simulink model "SWC_FDC_type"  (R2021b)
settings: Solver=FixedStepDiscrete  StartTime=0.0  StopTime=10.0  FixedStep=0.001  RelTol=1e-3
values from neighbouring files (symbols this model uses):
  DID_VCUKey = uint16(0x0202)    [vcu_local_hdr.m]
  DID_XWD = uint16(513)    [vcu_local_hdr.m]
  DIDLen_APSFunConfig = uint16(16)    [vcu_local_hdr.m]
  DIDLen_AutoLock = uint16(1)    [vcu_local_hdr.m]
  DIDLen_DKCKey = uint16(8)    [vcu_local_hdr.m]
  DIDLen_DRLDis = uint16(1)    [vcu_local_hdr.m]
  DIDLen_DynoMode = uint16(1)    [vcu_local_hdr.m]
  DIDLen_FMHTimer = uint16(1)    [vcu_local_hdr.m]
  DIDLen_LFLowPresThre = uint16(1)    [vcu_local_hdr.m]
  DIDLen_LFSensorID = uint16(4)    [vcu_local_hdr.m]
  DIDLen_LRLowPresThre = uint16(1)    [vcu_local_hdr.m]
  DIDLen_LRSensorID = uint16(4)    [vcu_local_hdr.m]
  DIDLen_RFLowPresThre = uint16(1)    [vcu_local_hdr.m]
  DIDLen_RFSensorID = uint16(4)    [vcu_local_hdr.m]
  DIDLen_RRLowPresThre = uint16(1)    [vcu_local_hdr.m]
  DIDLen_RRSensorID = uint16(4)    [vcu_local_hdr.m]
  DIDLen_SensorMode = uint16(1)    [vcu_local_hdr.m]
  DIDLen_TireSize = uint16(16)    [vcu_local_hdr.m]
  DIDLen_TPMSLearnSta = uint16(1)    [vcu_local_hdr.m]
  DIDLen_TurnLampFLThreCurr = uint16(1)    [vcu_local_hdr.m]
  DIDLen_TurnLampFRThreCurr = uint16(1)    [vcu_local_hdr.m]
  DIDLen_TurnLampRLThreCurr = uint16(1)    [vcu_local_hdr.m]
  DIDLen_TurnLampRRThreCurr = uint16(1)    [vcu_local_hdr.m]
  DIDLen_USSConfig = uint16(16)    [vcu_local_hdr.m]
  DIDLen_WhlPres = uint16(4)    [vcu_local_hdr.m]
  DIDLen_WhlSensorBattSta = uint16(1)    [vcu_local_hdr.m]
  DIDLen_WhlTmp = uint16(4)    [vcu_local_hdr.m]
  DIDLen_XWDMode = uint16(1)    [vcu_local_hdr.m]
  DIDNum_APSFunConfig = uint16(0x0903)    [vcu_local_hdr.m]
  DIDNum_AutoLock = uint16(0x0306)    [vcu_local_hdr.m]
  DIDNum_DKCKey = uint16(0x0202)    [vcu_local_hdr.m]
  DIDNum_DRLDis = uint16(0x0307)    [vcu_local_hdr.m]
  DIDNum_DynoMode = uint16(0x0203)    [vcu_local_hdr.m]
  DIDNum_FMHTimer = uint16(0x0305)    [vcu_local_hdr.m]
  DIDNum_LFLowPresThre = uint16(0x0B08)    [vcu_local_hdr.m]
  DIDNum_LFSensorID = uint16(0x0B01)    [vcu_local_hdr.m]
  DIDNum_LRLowPresThre = uint16(0x0B0A)    [vcu_local_hdr.m]
  DIDNum_LRSensorID = uint16(0x0B03)    [vcu_local_hdr.m]
  DIDNum_RFLowPresThre = uint16(0x0B09)    [vcu_local_hdr.m]
  DIDNum_RFSensorID = uint16(0x0B02)    [vcu_local_hdr.m]
  DIDNum_RRLowPresThre = uint16(0x0B0B)    [vcu_local_hdr.m]
  DIDNum_RRSensorID = uint16(0x0B04)    [vcu_local_hdr.m]
  DIDNum_SensorMode = uint16(0x0B0C)    [vcu_local_hdr.m]
  DIDNum_TireSize = uint16(0x0902)    [vcu_local_hdr.m]
  DIDNum_TPMSLearnSta = uint16(0x0B0D)    [vcu_local_hdr.m]
  DIDNum_TurnLampFLThreCurr = uint16(0x0303)    [vcu_local_hdr.m]
  DIDNum_TurnLampFRThreCurr = uint16(0x0301)    [vcu_local_hdr.m]
  DIDNum_TurnLampRLThreCurr = uint16(0x0304)    [vcu_local_hdr.m]
  DIDNum_TurnLampRRThreCurr = uint16(0x0302)    [vcu_local_hdr.m]
  DIDNum_USSConfig = uint16(0x0901)    [vcu_local_hdr.m]
  DIDNum_WhlPres = uint16(0x0B05)    [vcu_local_hdr.m]
  DIDNum_WhlSensorBattSta = uint16(0x0B07)    [vcu_local_hdr.m]
  DIDNum_WhlTmp = uint16(0x0B06)    [vcu_local_hdr.m]
  DIDNum_XWDMode = uint16(0x0201)    [vcu_local_hdr.m]
  DIDVCUKeyLength = uint16(8)    [vcu_local_hdr.m]
  ENUM_DRIVETRAIN_AWD = uint8(  2  )    [vcu_local_hdr.m]
  ENUM_DRIVETRAIN_FWD = uint8(  1  )    [vcu_local_hdr.m]
  ENUM_DRIVETRAIN_RWD = uint8(  0  )    [vcu_local_hdr.m]
  ENUM_TPMSLearnStatus_LEARNED = uint8(  1  )    [vcu_local_hdr.m]
  ENUM_TPMSLearnStatus_LEARNFAIL = uint8(  2  )    [vcu_local_hdr.m]
  ENUM_TPMSLearnStatus_NOTLEARN = uint8(  0  )    [vcu_local_hdr.m]
  ENUM_TPMSSTA_FAT = uint8(  8  )    [vcu_local_hdr.m]
  ENUM_TPMSSTA_LOWBATTERY = uint8(  2  )    [vcu_local_hdr.m]
  FALSE = boolean( 0 )    [vcu_local_hdr.m]
  ONE_INT = uint8(1)    [vcu_local_hdr.m]
  P_boolean = 0.0    [APPTypes.sldd]
  TRUE = boolean( 1 )    [vcu_local_hdr.m]
  ZERO_FLOAT = single(0)    [vcu_local_hdr.m]
  ZERO_INT = uint8(0)    [vcu_local_hdr.m]
undefined symbols (not defined in the file or in its folder): f32_ApsOutVehSpdSig, KHAL_DKCDecryptEnable_flg_ovrdflg, KHAL_DKCDecryptEnable_flg_ovrdval, KHAL_RandomNumberY1_enum, KHAL_RandomNumberY2_enum, KHAL_RandomNumberY_ovrdflg, KHAL_TPMSRESBUTT_flg_ovrdflg, KHAL_TPMSRESBUTT_flg_ovrdval, R_DIDWriteCDD_CSOP_DIDSet_APSFunConfig, R_DIDWriteCDD_CSOP_DIDSet_AutoLock, R_DIDWriteCDD_CSOP_DIDSet_DKCKey, R_DIDWriteCDD_CSOP_DIDSet_DRLDis, R_DIDWriteCDD_CSOP_DIDSet_DynoMode, R_DIDWriteCDD_CSOP_DIDSet_FMHTimer, R_DIDWriteCDD_CSOP_DIDSet_LFLowPresThre, R_DIDWriteCDD_CSOP_DIDSet_LFSensorID, R_DIDWriteCDD_CSOP_DIDSet_LRLowPresThre, R_DIDWriteCDD_CSOP_DIDSet_LRSensorID, R_DIDWriteCDD_CSOP_DIDSet_RFLowPresThre, R_DIDWriteCDD_CSOP_DIDSet_RFSensorID, R_DIDWriteCDD_CSOP_DIDSet_RRLowPresThre, R_DIDWriteCDD_CSOP_DIDSet_RRSensorID, R_DIDWriteCDD_CSOP_DIDSet_SensorMode, R_DIDWriteCDD_CSOP_DIDSet_TireSize, R_DIDWriteCDD_CSOP_DIDSet_TPMSLearnSta, R_DIDWriteCDD_CSOP_DIDSet_TurnLampFLThreCurr, R_DIDWriteCDD_CSOP_DIDSet_TurnLampFRThreCurr, R_DIDWriteCDD_CSOP_DIDSet_TurnLampRLThreCurr, R_DIDWriteCDD_CSOP_DIDSet_TurnLampRRThreCurr, R_DIDWriteCDD_CSOP_DIDSet_USSConfig, R_DIDWriteCDD_CSOP_DIDSet_WhlPres, R_DIDWriteCDD_CSOP_DIDSet_WhlSensorBattSta, R_DIDWriteCDD_CSOP_DIDSet_WhlTmp, R_DIDWriteCDD_CSOP_DIDSet_XWDMode, R_E2E_CAN3_VCU1_CSOP_Write_CAN3_VCU1, R_E2E_CAN3_VCU1_toNIDEC_CSOP_Write_CAN3_VCU1_toNIDEC, R_E2E_CAN4_VCU1_CSOP_Write_CAN4_VCU1, R_FDCCDD_Inner_CSOP_FDC_AppCallSleep, R_HALINCDD_CSOP_PAS_Handler, R_HALINCDD_CSOP_UDS_Main, R_HALOUT_APS_CSOP_ApsOutput, R_HALOUTCDD_CSOP_AppNmStateReq, R_HALOUTCDD_CSOP_SetAcoreRebootCmdACK, R_HALOUTCDD_CSOP_SetSysPwrStat, R_HALOUTCDD_CSOP_SleepRequest, R_IOExpOUT_CDD_CSOP_IOExpSetVal, R_J1939_CAN1_CFGEM1_BAM_CSOP_Write_CAN1_CFGEM1_BAM, R_J1939_CAN1_CFGEM1_DT_CSOP_Write_CAN1_CFGEM1_DT, R_NVMReadCDD_Inner_NVM_ReadOperation, R_NVMWriteCDD_Inner_NVM_WriteOperation, R_UDSCDD_CSOP_DdmRestartOperationCycle, R_WDGCDD_CSOP_Call_Watchdog, R_WDGCDD_CSOP_Call_WDG_AppEnd, R_WDGCDD_CSOP_Call_WDG_AppStart, u16_DIDLen_APSFunConfig, u16_DIDLen_AutoLock, u16_DIDLen_DKCKey, u16_DIDLen_DRLDis, u16_DIDLen_DynoMode, u16_DIDLen_FMHTimer ... (+83)
libraries: simulink x215, FVT_lib x143, hcu_lib x19, hdlsllib x9, app x1, halin x1, halout x1, inp x1, outp x1
(part 4 of 13)

== system SWC_FDC_type/run_SWC_FDC_RxTx_5ms_sys/Subsystem3 ==
  BOUTP_outputs : Inport
  Enable : EnablePort
  Bus Selector3 : BusSelector  OutputSignals=VOUTP_PowerSta_enum,VOUTP_BrkPedalPos_pct,VOUTP_ActAPSPosn_pct,VOUTP_LFRawWhlSpeed_kph,VOUTP_RFRawWhlSpeed_kph,VOUTP_LRRawWhlSpeed_kph,VOUTP_RRRawWhlSpeed_kph,VOUTP_LFRawWhlSpeedV_flg,VOUTP_RFRawWhlSpeedV_flg,VOUTP_LRRawWhlSpeedV_flg,VOUTP_RRRawWhlSpeedV_flg,VOUTP_LFWhlRotDir_enum,VOUTP_RFWhlRotDir_enum,VOUTP_LRWhlRotDir_enum,VOUTP_RRWhlRotDir_enum,VOUTP_LFPulseCountV_flg,VOUTP_RFPulseCountV_flg,VOUTP_LRPulseCountV_flg,VOUTP_RRPulseCountV_flg,VOUTP_LFPulseCount_enum,VOUTP_RFPulseCount_enum,VOUTP_LRPulseCount_enum,VOUTP_RRPulseCount_enum,VOUTP_VehSpeedToAPM_kph,VOUTP_APSCtrlAvail_flg,VOUTP_ShifterHandleCmd_enum,VOUTP_DriIntend_enum,VOUTP_EPSAOIControl_enum,VOUTP_SASAngle_Deg,VOUTP_SASSpeed_degps,VOUTP_SASSpeedValid_flg,VOUTP_SASCAL_flg,VOUTP_SASV_flg,VOUTP_GRADE_Deg,VOUTP_YawRate_degps,VOUTP_LatAccel_Gps,VOUTP_LongAccel_Gps,VOUTP_MCPressure_bar,VOUTP_YawRateV_flg,VOUTP_LatAccelV_flg,VOUTP_LongAccelV_flg,VOUTP_MCPressureV_bar,VOUTP_BrkSwSta_flg,VOUTP_BrkSwV_flg,VOUTP_ESCStandstill_flg,VOUTP_ESCAPSSta_enum,VOUTP_EPBExtReleaseAvail_flg,VOUTP_EPBExtApplyAvail_flg,VOUTP_EPBErrSta_enum,VOUTP_EPBSta_enum,VOUTP_AVMparkingcancel_enum,VOUTP_AVMparkingexcute_enum,VOUTP_AVMParkingmode_enum,VOUTP_AVMErrSTA_flg,VOUTP_IVIStatus_flg,VOUTP_CAASSw_enum,VOUTP_IVIScreen_enum,VOUTP_VehSpeedToAPM_kph,VOUTP_ABSActive_flg,VOUTP_TCSActiveToAPM_flg,VOUTP_DriverSeatBeltCmd_flg,VOUTP_RFPressIndi_enum,VOUTP_LFPressIndi_enum,VOUTP_RRPressIndi_enum,VOUTP_LRPressIndi_enum,VOUTP_sigAmbAirT_C,VOUTP_VehSpeedToAPM_kph,VOUTP_VehSpeedToAPM_kph
  Bus Selector4 : BusSelector  OutputSignals=VOUTP_BrkPedalPosTimeOut_flg,VOUTP_LFRawWhlSpeedTimeOut_flg,VOUTP_RFRawWhlSpeedTimeOut_flg,VOUTP_LRRawWhlSpeedTimeOut_flg,VOUTP_RRRawWhlSpeedTimeOut_flg,VOUTP_LFRawWhlSpeedVTimeOut_flg,VOUTP_RFRawWhlSpeedVTimeOut_flg,VOUTP_LRRawWhlSpeedVTimeOut_flg,VOUTP_RRRawWhlSpeedVTimeOut_flg,VOUTP_LFWhlRotDirTimeOut_flg,VOUTP_RFWhlRotDirTimeOut_flg,VOUTP_LRWhlRotDirTimeOut_flg,VOUTP_RRWhlRotDirTimeOut_flg,VOUTP_LFPulseCountVTimeOut_flg,VOUTP_RFPulseCountVTimeOut_flg,VOUTP_LRPulseCountVTimeOut_flg,VOUTP_RRPulseCountVTimeOut_flg,VOUTP_LFPulseCountTimeOut_flg,VOUTP_RFPulseCountTimeOut_flg,VOUTP_LRPulseCountTimeOut_flg,VOUTP_RRPulseCountTimeOut_flg,VOUTP_ShifterHandleCmdTimeOut_flg,VOUTP_DriIntendTimeOut_flg,VOUTP_EPSAOIControlTimeOut_flg,VOUTP_SASAngleTimeOut_flg,VOUTP_SASSpeedTimeOut_flg,VOUTP_SASSpeedValidTimeOut_flg,VOUTP_SASCALTimeOut_flg,VOUTP_SASVTimeOut_flg,VOUTP_GRADETimeOut_flg,VOUTP_YawRateTimeOut_flg,VOUTP_LatAccelTimeOut_flg,VOUTP_LongAccelTimeOut_flg,VOUTP_MCPressureTimeOut_flg,VOUTP_YawRateVTimeOut_flg,VOUTP_LatAccelVTimeOut_flg,VOUTP_LongAccelVTimeOut_flg,VOUTP_MCPressureVTimeOut_flg,VOUTP_BrkSwStaTimeOut_flg,VOUTP_BrkSwVTimeOut_flg,VOUTP_ESCStandstillTimeOut_flg,VOUTP_ESCAPSStaTimeOut_flg,VOUTP_EPBExtReleaseAvailTimeOut_flg,VOUTP_EPBExtApplyAvailTimeOut_flg,VOUTP_EPBErrStaTimeOut_flg,VOUTP_EPBStaTimeOut_flg,VOUTP_AVMparkingcancelTimeOut_flg,VOUTP_AVMparkingexcuteTimeOut_flg,VOUTP_AVMParkingmodeTimeOut_flg,VOUTP_AVMErrSTATimeOut_flg,VOUTP_IVIStatusTimeOut_flg,VOUTP_CAASSwTimeOut_flg,VOUTP_IVIScreenTimeOut_flg,VOUTP_ABSActiveTimeOut_flg,VOUTP_TCSActiveTimeOut_flg,VOUTP_DriverSeatBeltCmdTimeOut_flg,VOUTP_RFPressIndi_enum,VOUTP_LFPressIndi_enum,VOUTP_RRPressIndi_enum,VOUTP_LRPressIndi_enum,VOUTP_sigAmbAirT_C
  Data Type Conversion{6..13,17..19,21..96,98..106,123} (97 alike) : DataTypeConversion  OutDataTypeStr=uint8
  Data Type Conversion{14..16,20} (4 alike) : DataTypeConversion  OutDataTypeStr=int16
  Data Type Conversion4 : DataTypeConversion  OutDataTypeStr=single
  Ground{,1..10} (11 alike) : Ground
  R_HALOUT_APS_CSOP_ApsSetData : FunctionCaller  FunctionPrototype=R_HALOUT_APS_CSOP_ApsSetData(u8_SetPwrSta,f32_SetBrkPedalPos,f32_SetActAPSPosn,f32_SetLF_RawWhlSpeed,f32_SetRF_RawWhlSpeed,f32_SetLR_RawWhlSpeed,f32_SetRR_RawWhlSpeed,u8_SetLF_RawWhlSpeed_V,u8_SetRF_RawWhlSpeed_V,u8_SetLR_RawWhlSpeed_V,u8_SetRR_RawWhlSpeed_V,u8_SetLF_WhlRotDir,u8_SetRF_WhlRotDir,u8_SetLR_WhlRotDir,u8_SetRR_WhlRotDir,u8_SetLF_PulseCount_V,u8_SetRF_PulseCount_V,u8_SetLR_PulseCount_V,u8_SetRR_PulseCount_V,s16_SetLF_PulseCount,s16_SetRF_PulseCount,s16_SetLR_PulseCount,s16_SetRR_PulseCount,u8_SetAPS_Active,u8_SetAPS_CtrlAvail,u8_SetShifter_Handle_Cmd,u8_SetDriIntend,u8_SetEPS_AOI_Control,f32_SetSAS_Angle,f32_SetSAS_Speed,u8_SetSAS_Speed_Valid,u8_SetSAS_CAL,u8_SetSAS_OK,f32_SetGRADE,f32_SetYawRate,f32_SetLatAccel,f32_SetLongAccel,f32_SetMCPressure,u8_SetYawRate_V,u8_SetLatAccel_V,u8_SetLongAccel_V,u8_SetMCPressure_V,u8_SetBrkSw_Sta,u8_SetBrkSw_V,u8_SetESC_Standstill,u8_SetESC_APS_Sta,u8_SetEPBExtReleaseAvail,u8_SetEPBExtApplyAvail,u8_SetEPBErrSta,u8_SetEPBSta,u8_SetAllDoorSW,u8_SetHoodSW,u8_SetTailgate_SW,u8_SetAVM_parking_cancel,u8_SetAVM_parking_excute,u8_SetAVM_Parking_mode,u8_SetAVM_Err_STA,u8_SetIVI_Status,u8_SetCAAS_Sw,u8_SetIVI_Screen,u8_SetCAAS_CtrlAvail,u8_SetABS_Active,u8_SetTCS_Active,u8_SetDriverSeatBeltCmd,u8_SetDrDoorSW,u8_SetPsDoorSW,u8_SetRLDoorSW,u8_SetRRDoorSW,u8_SetRFPressIndi,u8_SetLFPressIndi,u8_SetRRPressIndi,u8_SetLRPressIndi,f32_SetsigAmbAirT,f32_SetVehActSpd,u8_SetCAAS_Active)  InputArgumentSpecifications=uint8(1), single(1), single(1), single(1), single(1), single(1), single(1), uint8(1), uint8(1), uint8(1), uint8(1), uint8(1), uint8(1), uint8(1), uint8(1), uint8(1), uint8(1), uint8(1), uint8(1), int16(1), int16(1), int16(1), int16(1), uint8(1), uint8(1), uint8(1), uint8(1), uint8(1), single(1), single(1), uint8(1), uint8(1), uint8(1), single(1), single(1), single(1), single(1), single(1), uint8(1), uint8(1), uint8(1), uint8(1), uint8(1), uint8(1), uint8(1), uint8(1), uint8(1), uint8(1), uint8(1), uint8(1), uint8(1), uint8(1), uint8(1), uint8(1), uint8(1), uint8(1), uint8(1), uint8(1), uint8(1), uint8(1), uint8(1), uint8(1), uint8(1), uint8(1), uint8(1), uint8(1), uint8(1), uint8(1), uint8(1), uint8(1), uint8(1), uint8(1), single(1), single(1), uint8(1)
  R_HALOUT_APS_CSOP_ApsSetTimeout : FunctionCaller  FunctionPrototype=R_HALOUT_APS_CSOP_ApsSetTimeout(u8_SetBrkPedalPosTO,u8_SetLF_RawWhlSpeedTO,u8_SetRF_RawWhlSpeedTO,u8_SetLR_RawWhlSpeedTO,u8_SetRR_RawWhlSpeedTO,u8_SetLF_RawWhlSpeed_VTO,u8_SetRF_RawWhlSpeed_VTO,u8_SetLR_RawWhlSpeed_VTO,u8_SetRR_RawWhlSpeed_VTO,u8_SetLF_WhlRotDirTO,u8_SetRF_WhlRotDirTO,u8_SetLR_WhlRotDirTO,u8_SetRR_WhlRotDirTO,u8_SetLF_PulseCount_VTO,u8_SetRF_PulseCount_VTO,u8_SetLR_PulseCount_VTO,u8_SetRR_PulseCount_VTO,u8_SetLF_PulseCountTO,u8_SetRF_PulseCountTO,u8_SetLR_PulseCountTO,u8_SetRR_PulseCountTO,u8_SetShifter_Handle_CmdTO,u8_SetDriIntendTO,u8_SetEPS_AOI_ControlTO,u8_SetSAS_AngleTO,u8_SetSAS_SpeedTO,u8_SetSAS_Speed_ValidTO,u8_SetSAS_CALTO,u8_SetSAS_OKTO,u8_SetGRADETO,u8_SetYawRateTO,u8_SetLatAccelTO,u8_SetLongAccelTO,u8_SetMCPressureTO,u8_SetYawRate_VTO,u8_SetLatAccel_VTO,u8_SetLongAccel_VTO,u8_SetMCPressure_VTO,u8_SetBrkSw_StaTO,u8_SetBrkSw_VTO,u8_SetESC_StandstillTO,u8_SetESC_APS_StaTO,u8_SetEPBExtReleaseAvailTO,u8_SetEPBExtApplyAvailTO,u8_SetEPBErrStaTO,u8_SetEPBStaTO,u8_SetAVM_parking_cancelTO,u8_SetAVM_parking_excuteTO,u8_SetAVM_Parking_modeTO,u8_SetAVM_Err_STATO,u8_SetIVI_StatusTO,u8_SetCAAS_SwTO,u8_SetIVI_ScreenTO,u8_SetABS_ActiveTO,u8_SetTCS_ActiveTO,u8_SetDriverSeatBeltCmdTO,u8_SetRFPressIndiTO,u8_SetLFPressIndiTO,u8_SetRRPressIndiTO,u8_SetLRPressIndiTO,u8_SetsigAmbAirTTO)  InputArgumentSpecifications=uint8(1), uint8(1), uint8(1), uint8(1), uint8(1), uint8(1), uint8(1), uint8(1), uint8(1), uint8(1), uint8(1), uint8(1), uint8(1), uint8(1), uint8(1), uint8(1), uint8(1), uint8(1), uint8(1), uint8(1), uint8(1), uint8(1), uint8(1), uint8(1), uint8(1), uint8(1), uint8(1), uint8(1), uint8(1), uint8(1), uint8(1), uint8(1), uint8(1), uint8(1), uint8(1), uint8(1), uint8(1), uint8(1), uint8(1), uint8(1), uint8(1), uint8(1), uint8(1), uint8(1), uint8(1), uint8(1), uint8(1), uint8(1), uint8(1), uint8(1), uint8(1), uint8(1), uint8(1), uint8(1), uint8(1), uint8(1), uint8(1), uint8(1), uint8(1), uint8(1), uint8(1)
  Terminator{1..9} (9 alike) : Terminator
  wires:
  Data Type Conversion75/1 -> R_HALOUT_APS_CSOP_ApsSetTimeout/33
  Bus Selector4/29 -> Data Type Conversion61/1  "<VOUTP_SASVTimeOut_flg>"
  Bus Selector3/45 -> Data Type Conversion30/1  "<VOUTP_ESCStandstill_flg>"
  Bus Selector4/41 -> Data Type Conversion73/1  "<VOUTP_ESCStandstillTimeOut_flg>"
  Data Type Conversion51/1 -> R_HALOUT_APS_CSOP_ApsSetTimeout/19
  Bus Selector4/1 -> Data Type Conversion80/1  "<VOUTP_BrkPedalPosTimeOut_flg>"
  Bus Selector4/10 -> Data Type Conversion42/1  "<VOUTP_LFWhlRotDirTimeOut_flg>"
  Data Type Conversion84/1 -> R_HALOUT_APS_CSOP_ApsSetTimeout/55
  Bus Selector3/48 -> Data Type Conversion32/1  "<VOUTP_EPBExtApplyAvail_flg>"
  Bus Selector3/43 -> Data Type Conversion28/1  "<VOUTP_BrkSwSta_flg>"
  Bus Selector3/56 -> R_HALOUT_APS_CSOP_ApsSetData/59  "<VOUTP_CAASSw_enum>"
  Bus Selector4/39 -> Data Type Conversion71/1  "<VOUTP_BrkSwStaTimeOut_flg>"
  Bus Selector3/39 -> Data Type Conversion24/1  "<VOUTP_YawRateV_flg>"
  Data Type Conversion123/1 -> R_HALOUT_APS_CSOP_ApsSetTimeout/2
  Bus Selector3/21 -> Data Type Conversion14/1  "<VOUTP_RFPulseCount_enum>"
  Bus Selector3/67 -> Terminator8/1  "<VOUTP_VehSpeedToAPM_kph>"
  Bus Selector3/54 -> Data Type Conversion36/1  "<VOUTP_AVMErrSTA_flg>"
  Bus Selector3/47 -> Data Type Conversion31/1  "<VOUTP_EPBExtReleaseAvail_flg>"
  Data Type Conversion82/1 -> R_HALOUT_APS_CSOP_ApsSetTimeout/47
  Bus Selector4/34 -> Data Type Conversion66/1  "<VOUTP_MCPressureTimeOut_flg>"
  Bus Selector4/42 -> Data Type Conversion76/1  "<VOUTP_ESCAPSStaTimeOut_flg>"
  Data Type Conversion85/1 -> R_HALOUT_APS_CSOP_ApsSetTimeout/49
  Bus Selector4/8 -> Data Type Conversion44/1  "<VOUTP_LRRawWhlSpeedVTimeOut_flg>"
  Bus Selector4/9 -> Data Type Conversion41/1  "<VOUTP_RRRawWhlSpeedVTimeOut_flg>"
  Bus Selector3/55 -> Data Type Conversion37/1  "<VOUTP_IVIStatus_flg>"
  Bus Selector4/46 -> Data Type Conversion79/1  "<VOUTP_EPBStaTimeOut_flg>"
  Bus Selector3/15 -> R_HALOUT_APS_CSOP_ApsSetData/15  "<VOUTP_RRWhlRotDir_enum>"
  Data Type Conversion35/1 -> R_HALOUT_APS_CSOP_ApsSetData/53
  Bus Selector4/37 -> Data Type Conversion69/1  "<VOUTP_LongAccelVTimeOut_flg>"
  Bus Selector4/17 -> Data Type Conversion49/1  "<VOUTP_RRPulseCountVTimeOut_flg>"
  Bus Selector3/34 -> R_HALOUT_APS_CSOP_ApsSetData/34  "<VOUTP_GRADE_Deg>"
  Ground9/1 -> Data Type Conversion96/1
  Bus Selector4/5 -> Data Type Conversion38/1  "<VOUTP_RRRawWhlSpeedTimeOut_flg>"
  Bus Selector4/2 -> Data Type Conversion123/1  "<VOUTP_LFRawWhlSpeedTimeOut_flg>"
  Data Type Conversion89/1 -> R_HALOUT_APS_CSOP_ApsSetTimeout/56
  Bus Selector4/11 -> Data Type Conversion43/1  "<VOUTP_RFWhlRotDirTimeOut_flg>"
  Bus Selector4/19 -> Data Type Conversion51/1  "<VOUTP_RFPulseCountTimeOut_flg>"
  Data Type Conversion60/1 -> R_HALOUT_APS_CSOP_ApsSetTimeout/27
  Data Type Conversion64/1 -> R_HALOUT_APS_CSOP_ApsSetTimeout/28
  Bus Selector3/20 -> Data Type Conversion20/1  "<VOUTP_LFPulseCount_enum>"
  Data Type Conversion21/1 -> R_HALOUT_APS_CSOP_ApsSetData/31
  Bus Selector4/33 -> Data Type Conversion75/1  "<VOUTP_LongAccelTimeOut_flg>"
  Bus Selector4/26 -> Data Type Conversion59/1  "<VOUTP_SASSpeedTimeOut_flg>"
  Data Type Conversion63/1 -> R_HALOUT_APS_CSOP_ApsSetTimeout/31
  Bus Selector4/40 -> Data Type Conversion72/1  "<VOUTP_BrkSwVTimeOut_flg>"
  Bus Selector4/56 -> Data Type Conversion89/1  "<VOUTP_DriverSeatBeltCmdTimeOut_flg>"
  Bus Selector4/48 -> Data Type Conversion83/1  "<VOUTP_AVMparkingexcuteTimeOut_flg>"
  Bus Selector4/6 -> Data Type Conversion39/1  "<VOUTP_LFRawWhlSpeedVTimeOut_flg>"
  Data Type Conversion26/1 -> R_HALOUT_APS_CSOP_ApsSetData/41
  Bus Selector4/60 -> Terminator4/1  "<VOUTP_LRPressIndi_enum>"
  Bus Selector4/51 -> Data Type Conversion86/1  "<VOUTP_IVIStatusTimeOut_flg>"
  Data Type Conversion103/1 -> R_HALOUT_APS_CSOP_ApsSetData/63
  Bus Selector4/57 -> Terminator1/1  "<VOUTP_RFPressIndi_enum>"
  Ground5/1 -> Data Type Conversion106/1
  Ground1/1 -> Data Type Conversion91/1
  Bus Selector4/27 -> Data Type Conversion60/1  "<VOUTP_SASSpeedValidTimeOut_flg>"
  Bus Selector3/66 -> R_HALOUT_APS_CSOP_ApsSetData/73  "<VOUTP_sigAmbAirT_C>"
  Data Type Conversion87/1 -> R_HALOUT_APS_CSOP_ApsSetTimeout/52
  Bus Selector4/13 -> Data Type Conversion55/1  "<VOUTP_RRWhlRotDirTimeOut_flg>"
  Data Type Conversion24/1 -> R_HALOUT_APS_CSOP_ApsSetData/39
  Data Type Conversion61/1 -> R_HALOUT_APS_CSOP_ApsSetTimeout/29
  Bus Selector4/7 -> Data Type Conversion40/1  "<VOUTP_RFRawWhlSpeedVTimeOut_flg>"
  Bus Selector4/35 -> Data Type Conversion67/1  "<VOUTP_YawRateVTimeOut_flg>"
  Bus Selector4/25 -> Data Type Conversion58/1  "<VOUTP_SASAngleTimeOut_flg>"
  Bus Selector3/49 -> R_HALOUT_APS_CSOP_ApsSetData/49  "<VOUTP_EPBErrSta_enum>"
  Data Type Conversion76/1 -> R_HALOUT_APS_CSOP_ApsSetTimeout/42
  Bus Selector4/55 -> Data Type Conversion84/1  "<VOUTP_TCSActiveTimeOut_flg>"
  Ground4/1 -> Data Type Conversion94/1
  Data Type Conversion39/1 -> R_HALOUT_APS_CSOP_ApsSetTimeout/6
  Bus Selector4/45 -> Data Type Conversion78/1  "<VOUTP_EPBErrStaTimeOut_flg>"
  Bus Selector4/12 -> Data Type Conversion45/1  "<VOUTP_LRWhlRotDirTimeOut_flg>"
  Bus Selector4/24 -> Data Type Conversion57/1  "<VOUTP_EPSAOIControlTimeOut_flg>"
  Data Type Conversion11/1 -> R_HALOUT_APS_CSOP_ApsSetData/17
  Bus Selector3/42 -> Data Type Conversion27/1  "<VOUTP_MCPressureV_bar>"
  Bus Selector4/20 -> Data Type Conversion52/1  "<VOUTP_LRPulseCountTimeOut_flg>"
  Bus Selector3/23 -> Data Type Conversion16/1  "<VOUTP_RRPulseCount_enum>"
  Bus Selector4/54 -> Data Type Conversion81/1  "<VOUTP_ABSActiveTimeOut_flg>"
  Bus Selector4/49 -> Data Type Conversion85/1  "<VOUTP_AVMParkingmodeTimeOut_flg>"
  Bus Selector4/22 -> Data Type Conversion56/1  "<VOUTP_ShifterHandleCmdTimeOut_flg>"
  Bus Selector4/38 -> Data Type Conversion74/1  "<VOUTP_MCPressureVTimeOut_flg>"
  Bus Selector4/50 -> Data Type Conversion95/1  "<VOUTP_AVMErrSTATimeOut_flg>"
  Bus Selector4/23 -> Data Type Conversion70/1  "<VOUTP_DriIntendTimeOut_flg>"
  Data Type Conversion25/1 -> R_HALOUT_APS_CSOP_ApsSetData/40
  Data Type Conversion92/1 -> R_HALOUT_APS_CSOP_ApsSetTimeout/60
  Bus Selector4/36 -> Data Type Conversion68/1  "<VOUTP_LatAccelVTimeOut_flg>"
  Bus Selector4/18 -> Data Type Conversion54/1  "<VOUTP_LFPulseCountTimeOut_flg>"
  Bus Selector4/15 -> Data Type Conversion47/1  "<VOUTP_RFPulseCountVTimeOut_flg>"
  Data Type Conversion9/1 -> R_HALOUT_APS_CSOP_ApsSetData/11
  Data Type Conversion10/1 -> R_HALOUT_APS_CSOP_ApsSetData/16
  Bus Selector4/21 -> Data Type Conversion53/1  "<VOUTP_RRPulseCountTimeOut_flg>"
  Bus Selector4/28 -> Data Type Conversion64/1  "<VOUTP_SASCALTimeOut_flg>"
  Data Type Conversion77/1 -> R_HALOUT_APS_CSOP_ApsSetTimeout/44
  Data Type Conversion23/1 -> R_HALOUT_APS_CSOP_ApsSetData/33
  Data Type Conversion93/1 -> R_HALOUT_APS_CSOP_ApsSetTimeout/59
  Data Type Conversion69/1 -> R_HALOUT_APS_CSOP_ApsSetTimeout/37
  Data Type Conversion46/1 -> R_HALOUT_APS_CSOP_ApsSetTimeout/14
  Data Type Conversion74/1 -> R_HALOUT_APS_CSOP_ApsSetTimeout/38
  Bus Selector3/25 -> Data Type Conversion18/1  "<VOUTP_APSCtrlAvail_flg>"
  Data Type Conversion62/1 -> R_HALOUT_APS_CSOP_ApsSetTimeout/30
  Data Type Conversion52/1 -> R_HALOUT_APS_CSOP_ApsSetTimeout/20
  Data Type Conversion71/1 -> R_HALOUT_APS_CSOP_ApsSetTimeout/39
  Data Type Conversion80/1 -> R_HALOUT_APS_CSOP_ApsSetTimeout/1
  Data Type Conversion43/1 -> R_HALOUT_APS_CSOP_ApsSetTimeout/11
  Bus Selector3/37 -> R_HALOUT_APS_CSOP_ApsSetData/37  "<VOUTP_LongAccel_Gps>"
  Bus Selector3/31 -> Data Type Conversion21/1  "<VOUTP_SASSpeedValid_flg>"
  Data Type Conversion86/1 -> R_HALOUT_APS_CSOP_ApsSetTimeout/51
  Data Type Conversion65/1 -> R_HALOUT_APS_CSOP_ApsSetTimeout/32
  Bus Selector3/53 -> R_HALOUT_APS_CSOP_ApsSetData/56  "<VOUTP_AVMParkingmode_enum>"
  Data Type Conversion32/1 -> R_HALOUT_APS_CSOP_ApsSetData/48
  Data Type Conversion106/1 -> R_HALOUT_APS_CSOP_ApsSetTimeout/57
  Bus Selector3/28 -> R_HALOUT_APS_CSOP_ApsSetData/28  "<VOUTP_EPSAOIControl_enum>"
  Data Type Conversion91/1 -> R_HALOUT_APS_CSOP_ApsSetTimeout/61
  Data Type Conversion70/1 -> R_HALOUT_APS_CSOP_ApsSetTimeout/23
  Data Type Conversion102/1 -> R_HALOUT_APS_CSOP_ApsSetData/64
  Data Type Conversion22/1 -> R_HALOUT_APS_CSOP_ApsSetData/32
  Data Type Conversion58/1 -> R_HALOUT_APS_CSOP_ApsSetTimeout/25
  Data Type Conversion66/1 -> R_HALOUT_APS_CSOP_ApsSetTimeout/34
  Data Type Conversion95/1 -> R_HALOUT_APS_CSOP_ApsSetTimeout/50
  Data Type Conversion42/1 -> R_HALOUT_APS_CSOP_ApsSetTimeout/10
  Data Type Conversion94/1 -> R_HALOUT_APS_CSOP_ApsSetTimeout/58
  Bus Selector4/30 -> Data Type Conversion62/1  "<VOUTP_GRADETimeOut_flg>"
  Data Type Conversion48/1 -> R_HALOUT_APS_CSOP_ApsSetTimeout/16
  Data Type Conversion81/1 -> R_HALOUT_APS_CSOP_ApsSetTimeout/54
  Data Type Conversion83/1 -> R_HALOUT_APS_CSOP_ApsSetTimeout/48
  Data Type Conversion15/1 -> R_HALOUT_APS_CSOP_ApsSetData/22
  Bus Selector3/16 -> Data Type Conversion10/1  "<VOUTP_LFPulseCountV_flg>"
  [BOUTP_outputs] -> Bus Selector3/1
  Bus Selector3/59 -> Data Type Conversion104/1  "<VOUTP_ABSActive_flg>"
  Bus Selector3/10 -> Data Type Conversion8/1  "<VOUTP_LRRawWhlSpeedV_flg>"
  Bus Selector3/51 -> R_HALOUT_APS_CSOP_ApsSetData/54  "<VOUTP_AVMparkingcancel_enum>"
  Bus Selector3/17 -> Data Type Conversion11/1  "<VOUTP_RFPulseCountV_flg>"
  Bus Selector3/14 -> R_HALOUT_APS_CSOP_ApsSetData/14  "<VOUTP_LRWhlRotDir_enum>"
  Ground6/1 -> Data Type Conversion17/1
  Data Type Conversion30/1 -> R_HALOUT_APS_CSOP_ApsSetData/45
  Bus Selector3/68 -> Terminator9/1  "<VOUTP_VehSpeedToAPM_kph>"
  Ground7/1 -> Data Type Conversion105/1
  Data Type Conversion55/1 -> R_HALOUT_APS_CSOP_ApsSetTimeout/13
  Bus Selector3/18 -> Data Type Conversion12/1  "<VOUTP_LRPulseCountV_flg>"
  Bus Selector3/41 -> Data Type Conversion26/1  "<VOUTP_LongAccelV_flg>"
  Bus Selector3/1 -> R_HALOUT_APS_CSOP_ApsSetData/1  "<VOUTP_PowerSta_enum>"
  Data Type Conversion8/1 -> R_HALOUT_APS_CSOP_ApsSetData/10
  Bus Selector3/60 -> Data Type Conversion103/1  "<VOUTP_TCSActiveToAPM_flg>"
  Bus Selector3/19 -> Data Type Conversion13/1  "<VOUTP_RRPulseCountV_flg>"
  Bus Selector3/32 -> Data Type Conversion22/1  "<VOUTP_SASCAL_flg>"
  Ground2/1 -> Data Type Conversion92/1
  Bus Selector4/3 -> Data Type Conversion50/1  "<VOUTP_RFRawWhlSpeedTimeOut_flg>"
  Data Type Conversion54/1 -> R_HALOUT_APS_CSOP_ApsSetTimeout/18
  Bus Selector4/47 -> Data Type Conversion82/1  "<VOUTP_AVMparkingcancelTimeOut_flg>"
  Bus Selector4/31 -> Data Type Conversion63/1  "<VOUTP_YawRateTimeOut_flg>"
  [BOUTP_outputs] -> Bus Selector4/1
  Bus Selector3/62 -> R_HALOUT_APS_CSOP_ApsSetData/69  "<VOUTP_RFPressIndi_enum>"
  Ground3/1 -> Data Type Conversion93/1
  Bus Selector4/14 -> Data Type Conversion46/1  "<VOUTP_LFPulseCountVTimeOut_flg>"
  Bus Selector4/16 -> Data Type Conversion48/1  "<VOUTP_LRPulseCountVTimeOut_flg>"
  Bus Selector3/8 -> Data Type Conversion6/1  "<VOUTP_LFRawWhlSpeedV_flg>"
  Bus Selector4/32 -> Data Type Conversion65/1  "<VOUTP_LatAccelTimeOut_flg>"
  Bus Selector4/52 -> Data Type Conversion87/1  "<VOUTP_CAASSwTimeOut_flg>"
  Bus Selector4/53 -> Data Type Conversion88/1  "<VOUTP_IVIScreenTimeOut_flg>"
  Data Type Conversion49/1 -> R_HALOUT_APS_CSOP_ApsSetTimeout/17
  Data Type Conversion6/1 -> R_HALOUT_APS_CSOP_ApsSetData/8
  Bus Selector4/4 -> Data Type Conversion19/1  "<VOUTP_LRRawWhlSpeedTimeOut_flg>"
  Bus Selector4/44 -> Data Type Conversion77/1  "<VOUTP_EPBExtApplyAvailTimeOut_flg>"
  Bus Selector4/58 -> Terminator2/1  "<VOUTP_LFPressIndi_enum>"
  Data Type Conversion34/1 -> R_HALOUT_APS_CSOP_ApsSetData/52
  Data Type Conversion88/1 -> R_HALOUT_APS_CSOP_ApsSetTimeout/53
  Bus Selector4/59 -> Terminator3/1  "<VOUTP_RRPressIndi_enum>"
  Data Type Conversion79/1 -> R_HALOUT_APS_CSOP_ApsSetTimeout/46
  Bus Selector4/61 -> Terminator5/1  "<VOUTP_sigAmbAirT_C>"
  Bus Selector4/43 -> Data Type Conversion90/1  "<VOUTP_EPBExtReleaseAvailTimeOut_flg>"
  Data Type Conversion67/1 -> R_HALOUT_APS_CSOP_ApsSetTimeout/35
  Data Type Conversion18/1 -> R_HALOUT_APS_CSOP_ApsSetData/25
  Data Type Conversion59/1 -> R_HALOUT_APS_CSOP_ApsSetTimeout/26
  Bus Selector3/58 -> Terminator7/1  "<VOUTP_VehSpeedToAPM_kph>"
  Bus Selector3/22 -> Data Type Conversion15/1  "<VOUTP_LRPulseCount_enum>"
  Bus Selector3/44 -> Data Type Conversion29/1  "<VOUTP_BrkSwV_flg>"
  Bus Selector3/29 -> R_HALOUT_APS_CSOP_ApsSetData/29  "<VOUTP_SASAngle_Deg>"
  Bus Selector3/61 -> Data Type Conversion102/1  "<VOUTP_DriverSeatBeltCmd_flg>"
  Bus Selector3/33 -> Data Type Conversion23/1  "<VOUTP_SASV_flg>"
  Bus Selector3/40 -> Data Type Conversion25/1  "<VOUTP_LatAccelV_flg>"
  Bus Selector3/9 -> Data Type Conversion7/1  "<VOUTP_RFRawWhlSpeedV_flg>"
  Data Type Conversion47/1 -> R_HALOUT_APS_CSOP_ApsSetTimeout/15
  Ground8/1 -> Data Type Conversion4/1
  Bus Selector3/24 -> Terminator6/1  "<VOUTP_VehSpeedToAPM_kph>"
  Bus Selector3/5 -> R_HALOUT_APS_CSOP_ApsSetData/5  "<VOUTP_RFRawWhlSpeed_kph>"
  Bus Selector3/11 -> Data Type Conversion9/1  "<VOUTP_RRRawWhlSpeedV_flg>"
  Data Type Conversion68/1 -> R_HALOUT_APS_CSOP_ApsSetTimeout/36
  Data Type Conversion57/1 -> R_HALOUT_APS_CSOP_ApsSetTimeout/24
  Data Type Conversion78/1 -> R_HALOUT_APS_CSOP_ApsSetTimeout/45
  Data Type Conversion38/1 -> R_HALOUT_APS_CSOP_ApsSetTimeout/5
  Data Type Conversion40/1 -> R_HALOUT_APS_CSOP_ApsSetTimeout/7
  Data Type Conversion19/1 -> R_HALOUT_APS_CSOP_ApsSetTimeout/4
  Data Type Conversion41/1 -> R_HALOUT_APS_CSOP_ApsSetTimeout/9
  Bus Selector3/63 -> R_HALOUT_APS_CSOP_ApsSetData/70  "<VOUTP_LFPressIndi_enum>"
  Data Type Conversion50/1 -> R_HALOUT_APS_CSOP_ApsSetTimeout/3
  Data Type Conversion44/1 -> R_HALOUT_APS_CSOP_ApsSetTimeout/8
  Data Type Conversion53/1 -> R_HALOUT_APS_CSOP_ApsSetTimeout/21
  Data Type Conversion56/1 -> R_HALOUT_APS_CSOP_ApsSetTimeout/22
  Data Type Conversion45/1 -> R_HALOUT_APS_CSOP_ApsSetTimeout/12
  Data Type Conversion72/1 -> R_HALOUT_APS_CSOP_ApsSetTimeout/40
  Data Type Conversion73/1 -> R_HALOUT_APS_CSOP_ApsSetTimeout/41
  Data Type Conversion90/1 -> R_HALOUT_APS_CSOP_ApsSetTimeout/43
  Data Type Conversion31/1 -> R_HALOUT_APS_CSOP_ApsSetData/47
  Data Type Conversion96/1 -> R_HALOUT_APS_CSOP_ApsSetData/75
  Bus Selector3/46 -> R_HALOUT_APS_CSOP_ApsSetData/46  "<VOUTP_ESCAPSSta_enum>"
  Bus Selector3/50 -> R_HALOUT_APS_CSOP_ApsSetData/50  "<VOUTP_EPBSta_enum>"
  Data Type Conversion27/1 -> R_HALOUT_APS_CSOP_ApsSetData/42
  Data Type Conversion104/1 -> R_HALOUT_APS_CSOP_ApsSetData/62
  Bus Selector3/57 -> R_HALOUT_APS_CSOP_ApsSetData/60  "<VOUTP_IVIScreen_enum>"
  Data Type Conversion100/1 -> R_HALOUT_APS_CSOP_ApsSetData/66
  Bus Selector3/64 -> R_HALOUT_APS_CSOP_ApsSetData/71  "<VOUTP_RRPressIndi_enum>"
  Data Type Conversion37/1 -> R_HALOUT_APS_CSOP_ApsSetData/58
  Data Type Conversion36/1 -> R_HALOUT_APS_CSOP_ApsSetData/57
  Bus Selector3/65 -> R_HALOUT_APS_CSOP_ApsSetData/72  "<VOUTP_LRPressIndi_enum>"
  Data Type Conversion7/1 -> R_HALOUT_APS_CSOP_ApsSetData/9
  Data Type Conversion4/1 -> R_HALOUT_APS_CSOP_ApsSetData/74
  Bus Selector3/27 -> R_HALOUT_APS_CSOP_ApsSetData/27  "<VOUTP_DriIntend_enum>"
  Bus Selector3/36 -> R_HALOUT_APS_CSOP_ApsSetData/36  "<VOUTP_LatAccel_Gps>"
  Data Type Conversion33/1 -> R_HALOUT_APS_CSOP_ApsSetData/51
  Bus Selector3/26 -> R_HALOUT_APS_CSOP_ApsSetData/26  "<VOUTP_ShifterHandleCmd_enum>"
  Data Type Conversion29/1 -> R_HALOUT_APS_CSOP_ApsSetData/44
  Data Type Conversion16/1 -> R_HALOUT_APS_CSOP_ApsSetData/23
  Data Type Conversion99/1 -> R_HALOUT_APS_CSOP_ApsSetData/67
  Data Type Conversion105/1 -> R_HALOUT_APS_CSOP_ApsSetData/61
  Data Type Conversion98/1 -> R_HALOUT_APS_CSOP_ApsSetData/68
  Bus Selector3/12 -> R_HALOUT_APS_CSOP_ApsSetData/12  "<VOUTP_LFWhlRotDir_enum>"
  Data Type Conversion101/1 -> R_HALOUT_APS_CSOP_ApsSetData/65
  Data Type Conversion28/1 -> R_HALOUT_APS_CSOP_ApsSetData/43
  Bus Selector3/38 -> R_HALOUT_APS_CSOP_ApsSetData/38  "<VOUTP_MCPressure_bar>"
  Bus Selector3/52 -> R_HALOUT_APS_CSOP_ApsSetData/55  "<VOUTP_AVMparkingexcute_enum>"
  Bus Selector3/4 -> R_HALOUT_APS_CSOP_ApsSetData/4  "<VOUTP_LFRawWhlSpeed_kph>"
  Bus Selector3/30 -> R_HALOUT_APS_CSOP_ApsSetData/30  "<VOUTP_SASSpeed_degps>"
  Bus Selector3/3 -> R_HALOUT_APS_CSOP_ApsSetData/3  "<VOUTP_ActAPSPosn_pct>"
  Bus Selector3/2 -> R_HALOUT_APS_CSOP_ApsSetData/2  "<VOUTP_BrkPedalPos_pct>"
  Bus Selector3/13 -> R_HALOUT_APS_CSOP_ApsSetData/13  "<VOUTP_RFWhlRotDir_enum>"
  Data Type Conversion13/1 -> R_HALOUT_APS_CSOP_ApsSetData/19
  Data Type Conversion14/1 -> R_HALOUT_APS_CSOP_ApsSetData/21
  Data Type Conversion12/1 -> R_HALOUT_APS_CSOP_ApsSetData/18
  Data Type Conversion17/1 -> R_HALOUT_APS_CSOP_ApsSetData/24
  Bus Selector3/6 -> R_HALOUT_APS_CSOP_ApsSetData/6  "<VOUTP_LRRawWhlSpeed_kph>"
  Bus Selector3/7 -> R_HALOUT_APS_CSOP_ApsSetData/7  "<VOUTP_RRRawWhlSpeed_kph>"
  Data Type Conversion20/1 -> R_HALOUT_APS_CSOP_ApsSetData/20
  Bus Selector3/35 -> R_HALOUT_APS_CSOP_ApsSetData/35  "<VOUTP_YawRate_degps>"
  BOUTP_outputs/1 -> [BOUTP_outputs]
  Ground/1 -> Data Type Conversion35/1, Data Type Conversion33/1, Data Type Conversion34/1
  Ground10/1 -> Data Type Conversion98/1, Data Type Conversion99/1, Data Type Conversion101/1, Data Type Conversion100/1

== system SWC_FDC_type/run_SWC_FDC_RxTx_5ms_sys/Subsystem4 ==
  Trig_BAM : Inport
  Trig_DT : Inport  Port=2
  function : TriggerPort  TriggerType=function-call  VariantControl=(inherit)
  Subsystem : Subsystem
  Subsystem1 : Subsystem
  wires:
  Trig_BAM/1 -> Subsystem/Enable
  Trig_DT/1 -> Subsystem1/Enable
